simulink model "original_model_two_loops"  (R2015b)
settings: Solver=ode45  StartTime=0.0  StopTime=280.0  RelTol=1e-3
values from neighbouring files (symbols this model uses):
  beta = 0.5    [fast_nullcline_winged_cusp.m]    (also in relay_model_bistability.m; relay_model_bistability2.m = 0.25)
  delta = 0.5    [fast_nullcline_winged_cusp.m]    (also in relay_model_bistability.m = 0.3; relay_model_bistability2.m = 0.3)
settings Model: Creator=ra428  LastModifiedBy=rajiv
settings DataIOCC: SaveFormat=Array
settings HardwareCC: ProdBitPerPointer=32  ProdLargestAtomicFloat=None  ProdIntDivRoundTo=Undefined  ProdEndianess=Unspecified  ProdWordSize=32  ProdHWDeviceType=32-bit Generic
settings GRTTargetCC: GeneratePreprocessorConditionals=Disable all
settings ConfigComp: CovModelRefEnable=Off

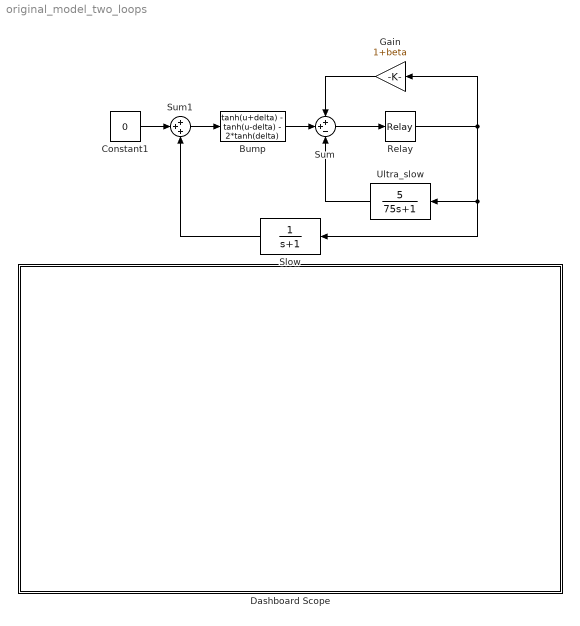
== system original_model_two_loops ==
  Bump : Fcn  Expr="tanh(u+delta) -  tanh(u-delta) - 2*tanh(delta)"
  Constant1 : Constant  Value=0
  Dashboard Scope : Subsystem  DialogController=hmiCreateDDGDialog  IsWebBlock=on  mask(MathWorksWebBlock){webBlockId=a72932a1-62b0-4401-931c-6d78c9731779, webBlockType=sdiscope, ShowInitialText=on, HMISrcModelName=original_model_two_loops}
      mask prompts: webBlockId "WebBlock Id"; webBlockType "WebBlock Type"; HMISrcModelName "Source Model"
      mask Help: helpview([docroot '/mapfiles/simulink.map'], 'hmi_scope')
      mask Display:
      | if strcmp(get_param(bdroot(gcb),'BlockDiagramType'), 'library')
      |     image([(matlabroot) '/toolbox/simulink/hmi/icons/DashboardScope.png']);
      | end
  Gain : Gain  Gain=1+beta
  Relay : Relay  OnSwitchValue=0  OffSwitchValue=0  OffOutputValue=-1
  Slow : TransferFcn  Denominator=[1 1]
  Sum : Sum  Inputs=++-
  Sum1 : Sum  Inputs=+++
  Ultra_slow : TransferFcn  Numerator=[5]  Denominator=[75 1]
  wires:
  Sum/1 -> Relay/1
  Gain/1 -> Sum/1
  Ultra_slow/1 -> Sum/3
  Constant1/1 -> Sum1/2
  Relay/1 -> Gain/1, Ultra_slow/1, Slow/1
  Slow/1 -> Sum1/3
  Bump/1 -> Sum/2
  Sum1/1 -> Bump/1

== system original_model_two_loops/Dashboard Scope ==
